simulink model "peter_spaceship_temp"  (R2024b)
settings: Solver=ode45  StartTime=0.0  StopTime=30  RelTol=1e-3  EnableMultiTasking=on
undefined symbols (not defined in the file): I, m
libraries: vrlib x2, sharedtransform x1, simulink_extras x1
Description:
  | Plane Take-Off with HUD Text
  | 
  | This model is a variant of the vrtkoff example that shows also how to display
  | signal values as text in the virtual scene and a simple Head-Up Display (HUD).
  | 
  | The text is sent to the virtual world as Simulink(R) string signal, composed from the numeric
  | input values using the format string (see sprintf for more information) and sent
  | to the 'string' field of the corresponding Text node in the world. Individual lines of
  | the MFString field are separated by the newline character in the format string.
  | 
  | The HUD behavior (maintaining constant relative position between the user and the
  | Text node) is achieved by defining a ProximitySensor that senses user position and
  | orientation as it navigates through the scene and routing this information to the translation
  | and rotation of HUD object - in this case a VRML Transform that contains the Text node.
settings Model: Creator=The MathWorks, Inc.  LastModifiedBy=peter
settings SolverCC: AlgebraicLoopSolver=TrustRegion
settings DataIOCC: LimitDataPoints=on  SaveFormat=Array  SaveOutput=off  SaveTime=off  ReturnWorkspaceOutputs=off  SignalLoggingName=logsOut
settings OptimizationCC: BlockReduction=off  BooleanDataType=off  ExpressionDepthLimit=2147483647  InitFltsAndDblsToZero=on  LifeSpan=inf
settings DebuggingCC: UnderspecifiedInitializationDetection=Classic  MergeDetectMultiDrivingBlocksExec=none  CheckExecutionContextPreStartOutputMsg=on  SignalResolutionControl=TryResolveAllWithWarning  MultiTaskDSMMsg=warning  MultiTaskCondExecSysMsg=none  FcnCallInpInsideContextMsg=warning  UnconnectedInputMsg=warning  UnconnectedOutputMsg=warning  UnconnectedLineMsg=warning  StateNameClashWarn=warning  SymbolicDimsDataTypeCodeGenerationDiagnostic=none  SFUnexpectedBacktrackingDiag=warning  SFNoUnconditionalDefaultTransitionDiag=warning  SFExecutionAtInitializationDiag=none  ArithmeticOperatorsInVariantConditions=warning
settings HardwareCC: ProdBitPerPointer=32  ProdBitPerSizeT=32  ProdBitPerPtrDiffT=32  ProdLargestAtomicFloat=None  ProdIntDivRoundTo=Undefined  ProdEndianess=Unspecified  ProdWordSize=32  ProdHWDeviceType=32-bit Generic  TargetUnknown=on
settings ModelReferenceCC: UpdateModelReferenceTargets=IfOutOfDate  EnableRefExpFcnMdlSchedulingChecks=on  PropagateSignalLabelsOutOfModel=off
settings SFSimCC: SimUseLocalCustomCode=off  CustomCodeUndefinedFunction=UseInterfaceOnly
settings RTWCC: RTWUseLocalCustomCode=off  GPUComputeCapability=3.5  DLArmComputeVersion=19.05
settings CodeAppCC: StateflowObjectComments=on
settings GRTTargetCC: TargetFcnLib=ansi_tfl_tmw.mat  TargetLangStandard=C89/C90 (ANSI)  CombineOutputUpdateFcns=off  GRTInterface=on
settings ConfigComp: CovMetricSettings=d  CovSaveCumulativeToWorkspaceVar=on  CovSaveSingleToWorkspaceVar=on  CovExternalEMLEnable=off  CovSFcnEnable=off

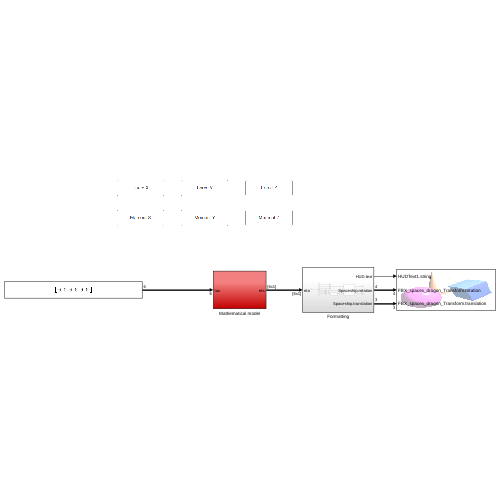
[thumbnail: Simulink's stored preview of the top-level diagram]
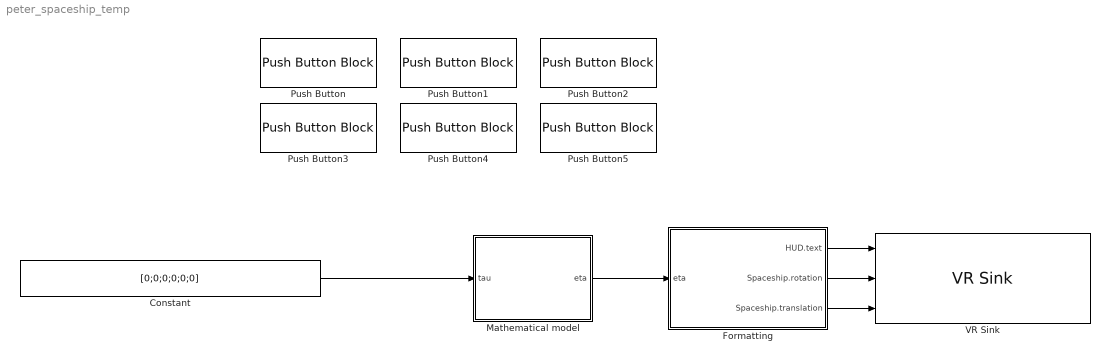
== system peter_spaceship_temp ==
  Constant : Constant  Value=[0;0;0;0;0;0]
  Formatting : Subsystem
  Mathematical model : Subsystem
  Push Button : PushButtonBlock  ButtonText=Force X  OnValue=100000  ButtonType=Latch  OffValue=0.000000
  Push Button1 : PushButtonBlock  ButtonText=Force Y  OnValue=100000  ButtonType=Latch  OffValue=0.000000
  Push Button2 : PushButtonBlock  ButtonText=Force Z  OnValue=-100000  ButtonType=Latch  OffValue=0.000000
  Push Button3 : PushButtonBlock  ButtonText=Moment X  OnValue=10000  ButtonType=Latch  OffValue=0.000000
  Push Button4 : PushButtonBlock  ButtonText=Moment Y  OnValue=10000  ButtonType=Latch  OffValue=0.000000
  Push Button5 : PushButtonBlock  ButtonText=Moment Z  OnValue=10000  ButtonType=Latch  OffValue=0.000000
  VR Sink : vrlib/VR Sink  InstantiateOnLoad=on  SampleTime=0.1  ViewEnable=on  RemoteChange=off  RemoteView=off  FieldsWritten=HUDText1.string.1.-1.1.char#FBX_spacex_dragon_Transform.rotation.4.1.1.double#FBX_spacex_dragon_Transform.translation.3.1.1.double  WorldFileName=spaceship_VR.x3d  WorldDescription=VR Spaceship Dragon  AutoView=off  VideoDimensions=[]  AllowVariableSize=off
  wires:
  Formatting/1(HUD.text) -> VR Sink/1
  Formatting/2(Spaceship.rotation) -> VR Sink/2
  Formatting/3(Spaceship.translation) -> VR Sink/3
  Mathematical model/1(eta) -> Formatting/1(eta)
  Constant/1 -> Mathematical model/1(tau)

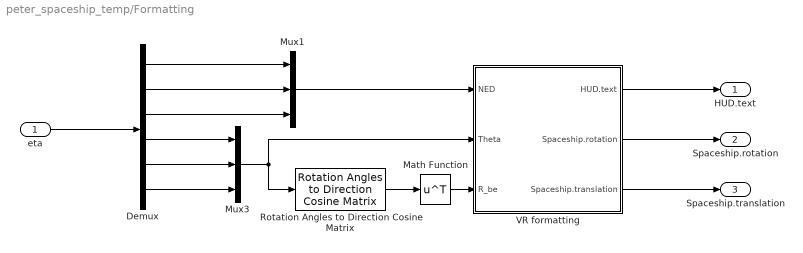
== system peter_spaceship_temp/Formatting ==
  eta : Inport
  Demux : Demux  Outputs=6
  Math Function : Math  Operator=transpose
  Mux1 : Mux  Inputs=3
  Mux3 : Mux  Inputs=3
  Rotation Angles to Direction Cosine Matrix : sharedtransform/Rotation Angles to Direction Cosine Matrix  rotationOrder=XYZ  aMode=aMode
  VR formatting : Subsystem
  HUD.text : Outport
  Spaceship.rotation : Outport  Port=2
  Spaceship.translation : Outport  Port=3
  wires:
  Demux/2 -> Mux1/2
  Demux/3 -> Mux1/3
  Mux1/1 -> VR formatting/1(NED)
  Demux/5 -> Mux3/2
  eta/1 -> Demux/1
  Demux/4 -> Mux3/1
  Demux/6 -> Mux3/3
  Math Function/1 -> VR formatting/3(R_be)
  Rotation Angles to Direction Cosine Matrix/1 -> Math Function/1
  Demux/1 -> Mux1/1
  VR formatting/1(HUD.text) -> HUD.text/1
  VR formatting/2(Spaceship.rotation) -> Spaceship.rotation/1
  VR formatting/3(Spaceship.translation) -> Spaceship.translation/1
  Mux3/1 -> Rotation Angles to Direction Cosine Matrix/1, VR formatting/2(Theta)

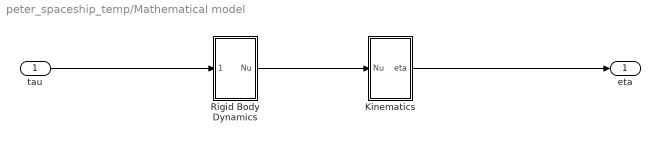
== system peter_spaceship_temp/Mathematical model ==
  tau : Inport
  Kinematics : Subsystem
  Rigid Body Dynamics : Subsystem
  eta : Outport
  wires:
  tau/1 -> Rigid Body Dynamics/1(Input)
  Kinematics/1(eta) -> eta/1
  Rigid Body Dynamics/1(Nu) -> Kinematics/1(Nu)

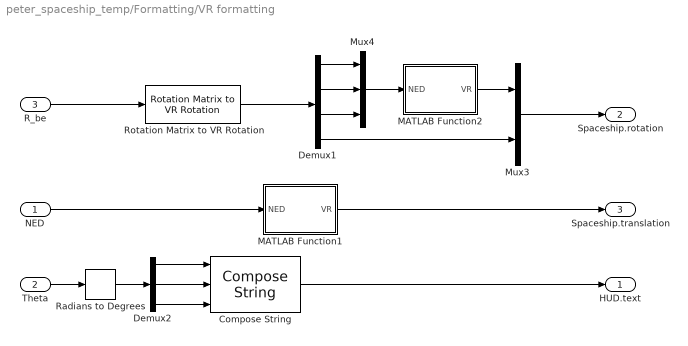
== system peter_spaceship_temp/Formatting/VR formatting ==
  NED : Inport
  Theta : Inport  Port=2
  R_be : Inport  Port=3
  Compose String : ComposeString  Format="'Roll    : %7.2f deg\\nPitch   : %7.2f deg\\nYaw     : %7.2f deg'"
  Demux1 : Demux
  Demux2 : Demux  Outputs=3
  MATLAB Function1 : MATLAB Function  TreatAsAtomicUnit=on
  MATLAB Function2 : MATLAB Function  TreatAsAtomicUnit=on
  Mux3 : Mux  Inputs=2
  Mux4 : Mux  Inputs=3
  Radians to Degrees : simulink_extras/Transformations/Radians to Degrees
  Rotation Matrix to VR Rotation : vrlib/Utilities/Rotation Matrix to VR Rotation  maxzero=1e-12
  HUD.text : Outport
  Spaceship.rotation : Outport  Port=2
  Spaceship.translation : Outport  Port=3
  wires:
  Rotation Matrix to VR Rotation/1 -> Demux1/1
  Mux3/1 -> Spaceship.rotation/1
  MATLAB Function2/1(VR) -> Mux3/1
  Mux4/1 -> MATLAB Function2/1(NED)
  Demux1/3 -> Mux4/3
  Demux1/1 -> Mux4/1
  Demux1/2 -> Mux4/2
  Demux1/4 -> Mux3/2
  NED/1 -> MATLAB Function1/1(NED)
  MATLAB Function1/1(VR) -> Spaceship.translation/1
  Demux2/1 -> Compose String/1
  Demux2/2 -> Compose String/2
  Demux2/3 -> Compose String/3
  Compose String/1 -> HUD.text/1
  Theta/1 -> Radians to Degrees/1
  R_be/1 -> Rotation Matrix to VR Rotation/1
  Radians to Degrees/1 -> Demux2/1

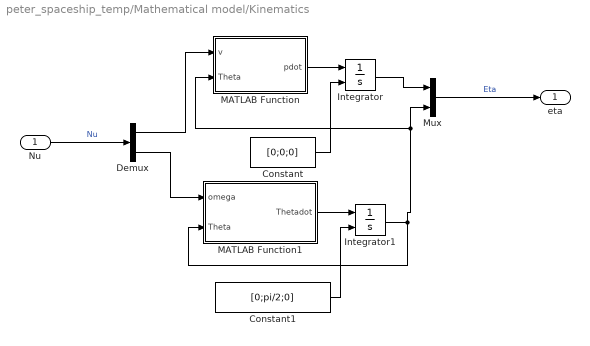
== system peter_spaceship_temp/Mathematical model/Kinematics ==
  Nu : Inport
  Constant : Constant  Value=[0;0;0]
  Constant1 : Constant  Value=[0;pi/2;0]
  Demux : Demux  Outputs=2
  Integrator : Integrator  InitialConditionSource=external
  Integrator1 : Integrator  InitialConditionSource=external
  MATLAB Function : MATLAB Function  TreatAsAtomicUnit=on
  MATLAB Function1 : MATLAB Function  TreatAsAtomicUnit=on
  Mux : Mux  Inputs=2
  eta : Outport
  wires:
  Mux/1 -> eta/1  "Eta"
  Nu/1 -> Demux/1  "Nu"
  Demux/1 -> MATLAB Function/1(v)
  MATLAB Function/1(pdot) -> Integrator/1
  Integrator/1 -> Mux/1
  MATLAB Function1/1(Thetadot) -> Integrator1/1
  Integrator1/1 -> Mux/2, MATLAB Function/2(Theta), MATLAB Function1/2(Theta)
  Demux/2 -> MATLAB Function1/1(omega)
  Constant/1 -> Integrator/2
  Constant1/1 -> Integrator1/2

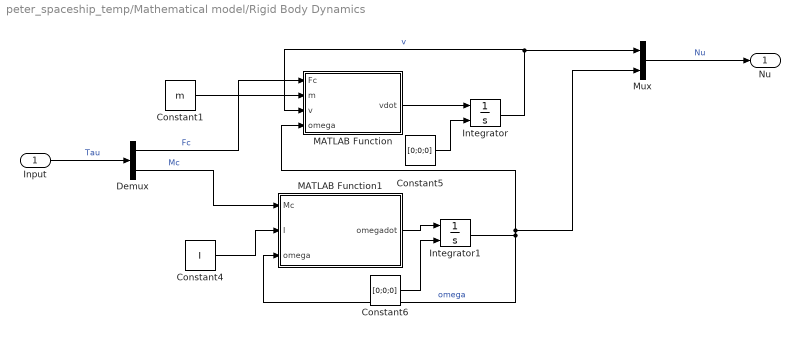
== system peter_spaceship_temp/Mathematical model/Rigid Body Dynamics ==
  Input : Inport
  Constant1 : Constant  Value=m
  Constant4 : Constant  Value=I
  Constant5 : Constant  Value=[0;0;0]
  Constant6 : Constant  Value=[0;0;0]
  Demux : Demux  Outputs=2
  Integrator : Integrator  InitialConditionSource=external
  Integrator1 : Integrator  InitialConditionSource=external
  MATLAB Function : MATLAB Function  TreatAsAtomicUnit=on
  MATLAB Function1 : MATLAB Function  TreatAsAtomicUnit=on
  Mux : Mux  Inputs=2
  Nu : Outport
  wires:
  MATLAB Function/1(vdot) -> Integrator/1
  MATLAB Function1/1(omegadot) -> Integrator1/1
  Constant4/1 -> MATLAB Function1/2(I)
  Integrator/1 -> Mux/1, MATLAB Function/3(v)  "v"
  Constant5/1 -> Integrator/2
  Constant1/1 -> MATLAB Function/2(m)
  Integrator1/1 -> MATLAB Function/4(omega), Mux/2, MATLAB Function1/3(omega)  "omega"
  Constant6/1 -> Integrator1/2
  Mux/1 -> Nu/1  "Nu"
  Input/1 -> Demux/1  "Tau"
  Demux/1 -> MATLAB Function/1(Fc)  "Fc"
  Demux/2 -> MATLAB Function1/1(Mc)  "Mc"

== matlab function peter_spaceship_temp/Mathematical model/Rigid Body Dynamics/MATLAB Function1 ==
  data: Mc input; omegadot output; I input; omega input
function omegadot = fcn(Mc, I, omega)
omegadot = inv(I)*(Mc - cross(omega, I*omega));

== matlab function peter_spaceship_temp/Mathematical model/Rigid Body Dynamics/MATLAB Function ==
  data: Fc input; vdot output; m input; v input; omega input
function vdot = fcn(Fc, m, v, omega)
vdot = 1/m * (Fc - cross(omega, m*v));

== matlab function peter_spaceship_temp/Mathematical model/Kinematics/MATLAB Function ==
  data: v input; pdot output; Theta input
function pdot = fcn(v, Theta)
    roll = Theta(1);
    pitch = Theta(2);
    yaw = Theta(3);
    
    rotation = Rz(yaw) * Ry(pitch) * Rx(roll);
    
    pdot = rotation * v;
end

function Rot = Rx(roll)
    Rot = [1,        0,         0;
           0,        cos(roll),  -sin(roll);
           0,        sin(roll),   cos(roll);];
end

function Rot = Ry(pitch)
    Rot = [cos(pitch),  0,    sin(pitch);
           0,           1,    0;
           -sin(pitch), 0     cos(pitch);];
end

function Rot = Rz(yaw)
    Rot = [cos(yaw), -sin(yaw), 0; 
           sin(yaw), cos(yaw),  0;
           0,        0,         1;];
end

== matlab function peter_spaceship_temp/Mathematical model/Kinematics/MATLAB Function1 ==
  data: omega input; Thetadot output; Theta input
function Thetadot = fcn(omega, Theta)
roll = Theta(1); %phi
pitch = Theta(2); %theta
yaw = Theta(3); %psi

Thetadot = Transformation(roll, pitch, yaw) * omega;
end

function mat = Transformation(roll, pitch, yaw)
    mat = [1,        sin(roll)*sin(pitch)/cos(pitch),   cos(roll)*sin(pitch)/cos(pitch);
           0,        cos(roll),                         -sin(roll);
           0,        sin(roll)/cos(pitch),              cos(roll)/cos(pitch);];
end

== matlab function peter_spaceship_temp/Formatting/VR formatting/MATLAB Function1 ==
  data: NED input; VR output
function VR = NED2VR(NED)

x = NED(1); % north
y = NED(2); % east 
z = NED(3); % down

VR = [ -y ; -z ; x ];

== matlab function peter_spaceship_temp/Formatting/VR formatting/MATLAB Function2 ==
  data: NED input; VR output
function VR = NED2VR(NED)

x = NED(1); % north
y = NED(2); % east 
z = NED(3); % down

VR = [ -y ; -z ; x ];
